simulink library "calculateReelOutSpeed"  (R2018a)
settings: Solver=VariableStepAuto  StartTime=0.0  StopTime=10.0  RelTol=1e-3
settings Model: Creator=mitch  LastModifiedBy=mitch

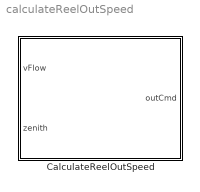
== system calculateReelOutSpeed ==
  CalculateReelOutSpeed : Subsystem

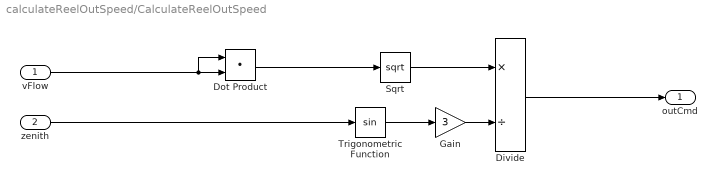
== system calculateReelOutSpeed/CalculateReelOutSpeed ==
  vFlow : Inport
  zenith : Inport  Port=2
  Divide : Product  Inputs=*/
  Dot Product : DotProduct  InputSameDT=on  OutDataTypeStr=Inherit: Inherit via internal rule
  Gain : Gain  Gain=3
  Sqrt : Sqrt  SaturateOnIntegerOverflow=on
  Trigonometric Function : Trigonometry
  outCmd : Outport
  wires:
  Sqrt/1 -> Divide/1
  Trigonometric Function/1 -> Gain/1
  Gain/1 -> Divide/2
  Divide/1 -> outCmd/1
  Dot Product/1 -> Sqrt/1
  vFlow/1 -> Dot Product/2, Dot Product/1
  zenith/1 -> Trigonometric Function/1
